simulink model "map_R2014a"  (R2014a)
settings: Solver=FixedStepDiscrete  StartTime=0  StopTime=300  FixedStep=0.5  RelTol=1e-3
PostLoadFcn:
  | , if any(exist('dsrtsu_mdlpostloadfcn', 'file') == [2, 3, 6]), try dsrtsu_mdlpostloadfcn('Execute', bdroot); catch fprintf('Error in PostLoadFcn (dsrtsu_mdlpostloadfcn) for model "%s":\n %s\n', bdroot, lasterr); end, end,
InitFcn:
  | load 'data/chi2_dat';
  | load 'data/innerLine_struct';
  | load 'data/middleLine_struct';
  | load 'data/outerLine_struct';
  | load 'data/innerLine';
  | load 'data/middleLine';
  | load 'data/outerLine';
  | load 'data/landmarks_patac_schimmel_ccw';
  | load 'data/patac_navi_array';
  | load 'data/sensor';
  | load 'data/map_struct';
  | addpath map_src
  | Integration_Parameter;
  | load 'TestData_001';
undefined symbols (not defined in the file or in its folder): chi2_dat, innerLine, landmarks_patac_schimmel_ccw, middleLine, outerLine, patac_navi_array
settings Model: DSRTSU_INTERNAL_RTI_VER=460  DSRTSU_INTERNAL_RTI_TYPE=rti1401  DSRTSU_INTERNAL_RTIFLEXRAYCONFIG=10  DSRTSU_INTERNAL_RTIFPGA=50  Creator=si8cwy  LastModifiedBy=Administrator
settings DataIOCC: SignalLoggingSaveFormat=ModelDataLogs
settings OptimizationCC: BlockReduction=off  ConditionallyExecuteInputs=off  OptimizeBlockIOStorage=off  BufferReuse=off  GlobalBufferReuse=off  ExpressionFolding=off  ExpressionDepthLimit=2147483647  LocalBlockOutputs=off  RollThreshold=100
settings DebuggingCC: MergeDetectMultiDrivingBlocksExec=error  MultiTaskDSMMsg=warning  MultiTaskCondExecSysMsg=none  FrameProcessingCompatibilityMsg=error  StateNameClashWarn=warning
settings HardwareCC: ProdIntDivRoundTo=Zero  ProdEndianess=BigEndian  ProdHWDeviceType=Generic->Custom  TargetIntDivRoundTo=Zero  TargetEndianess=BigEndian  TargetHWDeviceType=Generic->Custom
settings RTWCC: SystemTargetFile=rti1401.tlc  MakeCommand=make_rti  TemplateMakefile=rti1401.tmf  Description=dSPACE DS1401 Hardware Platform
settings STFCustomTargetCC: ParMdlRefBuildCompliant=on  ConcurrentExecutionCompliant=off  GeneratePreprocessorConditionals=Use local settings  SystemTargetFile=rti1401.tlc
settings GRTTargetCC: CompOptLevelCompliant=off  ConcurrentExecutionCompliant=off  GeneratePreprocessorConditionals=Use local settings  CombineOutputUpdateFcns=off  MatFileLogging=off  CPPClassGenCompliant=off  GRTInterface=on  ExtModeMexFile=noextcomm

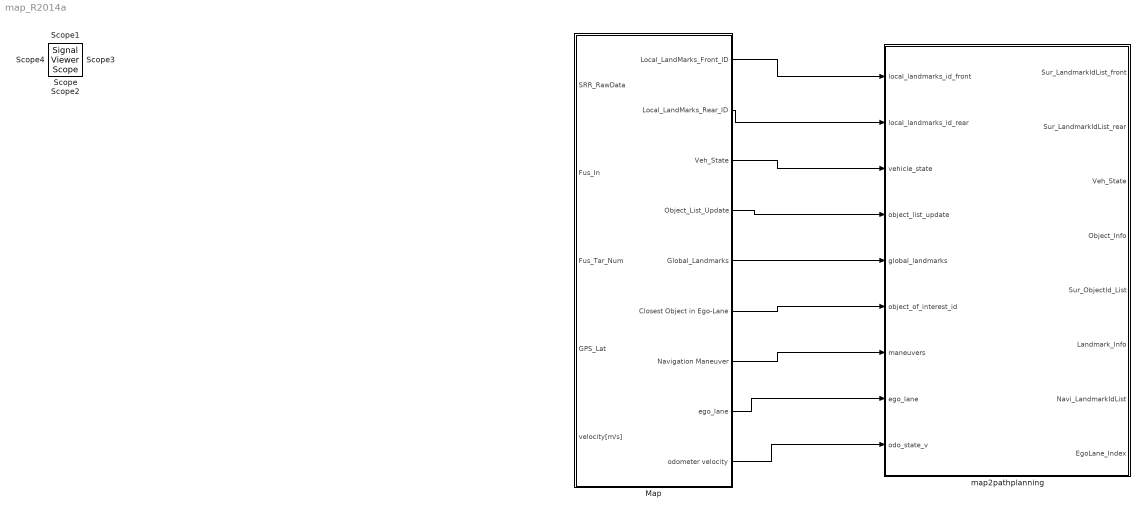
== system map_R2014a ==
  Map : Subsystem
  map2pathplanning : MATLAB Function  TreatAsAtomicUnit=on
      settings: PermitHierarchicalResolution=ParametersOnly
  Scope{,1..4} (5 alike) : SignalViewerScope  IOType=viewer  SampleTime=-1  ZoomMode=on
      Scope settings: TimeRange=auto  TickLabels=OneTimeTick  SaveToWorkspace=off  SaveName=ScopeData  YMin=-10  YMax=10  SampleInput=off
      Scope1 settings: TimeRange=auto  TickLabels=OneTimeTick  SaveToWorkspace=off  YMin=-10  YMax=10  SampleInput=off
      Scope2 settings: TimeRange=auto  TickLabels=OneTimeTick  SaveToWorkspace=off  SaveName=ScopeData2  YMin=-10  YMax=10  SampleInput=off
      Scope3 settings: TimeRange=auto  TickLabels=OneTimeTick  LimitDataPoints=on  SaveToWorkspace=off  SaveName=ScopeData3  YMin=-10  YMax=10  SampleInput=off
      Scope4 settings: TimeRange=auto  TickLabels=OneTimeTick  SaveToWorkspace=off  SaveName=ScopeData4  YMin=-10  YMax=10  SampleInput=off
  wires:
  Map/1(Local_LandMarks_Front_ID) -> map2pathplanning/1(local_landmarks_id_front)
  Map/3(Veh_State) -> map2pathplanning/3(vehicle_state)
  Map/4(Object_List_Update) -> map2pathplanning/4(object_list_update)
  Map/5("Global_Landmarks ") -> map2pathplanning/5(global_landmarks)
  Map/6(Closest Object in Ego-Lane) -> map2pathplanning/6(object_of_interest_id)
  Map/7(Navigation Maneuver) -> map2pathplanning/7(maneuvers)
  Map/9(odometer velocity) -> map2pathplanning/9(odo_state_v)
  Map/8(ego_lane) -> map2pathplanning/8(ego_lane)
  Map/2(Local_LandMarks_Rear_ID) -> map2pathplanning/2(local_landmarks_id_rear)

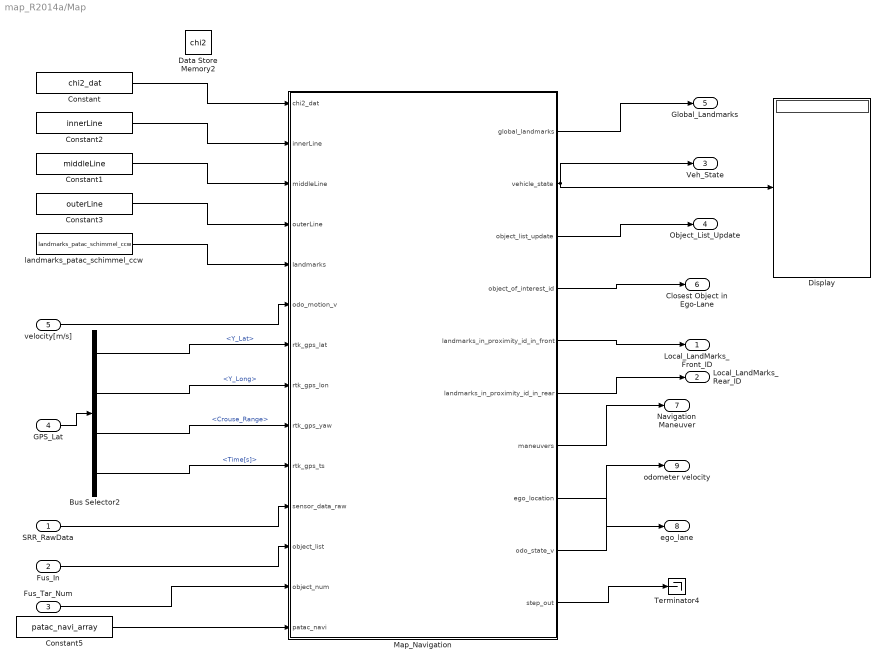
== system map_R2014a/Map ==
  SRR_RawData : Inport
  Fus_In : Inport  Port=2
  Fus_Tar_Num : Inport  Port=3
  GPS_Lat : Inport  Port=4
  velocity[m/s] : Inport  Port=5
  Bus Selector2 : BusSelector  OutputSignals=GPGLL.Y_Lat,GPGLL.Y_Long,GPHPR.Crouse_Range,GPGLL.Time[s]
  Constant : Constant  Value=chi2_dat
  Constant1 : Constant  Value=middleLine  OutDataTypeStr=Bus: middleLine_struct
  Constant2 : Constant  Value=innerLine  OutDataTypeStr=Bus: innerLine_struct
  Constant3 : Constant  Value=outerLine  OutDataTypeStr=Bus: outerLine_struct
  Constant5 : Constant  Value=patac_navi_array  OutDataTypeStr=double
  Data Store Memory2 : DataStoreMemory  DataStoreName=chi2  ReadBeforeWriteMsg=warning  WriteAfterWriteMsg=warning  WriteAfterReadMsg=warning  InitialValue=zeros(1,1000)  ShowAdditionalParam=off  OutDataTypeStr=double
  Display : Display
  Map_Navigation : MATLAB Function  TreatAsAtomicUnit=on
      settings: PermitHierarchicalResolution=ParametersOnly
  Terminator4 : Terminator
  landmarks_patac_schimmel_ccw : Constant  Value=landmarks_patac_schimmel_ccw  OutDataTypeStr=double
  Local_LandMarks_Front_ID : Outport
  Local_LandMarks_Rear_ID : Outport  Port=2
  Veh_State : Outport  Port=3
  Object_List_Update : Outport  Port=4
  "Global_Landmarks " : Outport  Port=5
  Closest Object in Ego-Lane : Outport  Port=6
  Navigation Maneuver : Outport  Port=7
  ego_lane : Outport  Port=8
  odometer velocity : Outport  Port=9
  wires:
  Map_Navigation/3(object_list_update) -> Object_List_Update/1
  Map_Navigation/2(vehicle_state) -> Veh_State/1, Display/1
  velocity[m/s]/1 -> Map_Navigation/6(odo_motion_v)
  GPS_Lat/1 -> Bus Selector2/1
  Bus Selector2/1 -> Map_Navigation/7(rtk_gps_lat)  "<Y_Lat>"
  Bus Selector2/2 -> Map_Navigation/8(rtk_gps_lon)  "<Y_Long>"
  Bus Selector2/3 -> Map_Navigation/9(rtk_gps_yaw)  "<Crouse_Range>"
  Bus Selector2/4 -> Map_Navigation/10(rtk_gps_ts)  "<Time[s]>"
  SRR_RawData/1 -> Map_Navigation/11(sensor_data_raw)
  Fus_In/1 -> Map_Navigation/12(object_list)
  Map_Navigation/4(object_of_interest_id) -> Closest Object in Ego-Lane/1
  Map_Navigation/7(maneuvers) -> Navigation Maneuver/1
  Constant/1 -> Map_Navigation/1(chi2_dat)
  Constant2/1 -> Map_Navigation/2(innerLine)
  Constant1/1 -> Map_Navigation/3(middleLine)
  Constant3/1 -> Map_Navigation/4(outerLine)
  landmarks_patac_schimmel_ccw/1 -> Map_Navigation/5(landmarks)
  Constant5/1 -> Map_Navigation/14(patac_navi)
  Map_Navigation/10(step_out) -> Terminator4/1
  Map_Navigation/9(odo_state_v) -> odometer velocity/1
  Map_Navigation/5(landmarks_in_proximity_id_in_front) -> Local_LandMarks_Front_ID/1
  Map_Navigation/1(global_landmarks) -> "Global_Landmarks "/1
  Map_Navigation/8(ego_location) -> ego_lane/1
  Map_Navigation/6(landmarks_in_proximity_id_in_rear) -> Local_LandMarks_Rear_ID/1
  Fus_Tar_Num/1 -> Map_Navigation/13(object_num)

== matlab function map_R2014a/Map/Map_Navigation ==
  data: global_landmarks output; vehicle_state output; object_list_update output; object_of_interest_id output; chi2_dat input; innerLine input; middleLine input; outerLine input; landmarks input; landmarks_in_proximity_id_in_front output [1..]; landmarks_in_proximity_id_in_rear output; odo_motion_v input; rtk_gps_lat input; rtk_gps_lon input; rtk_gps_yaw input; rtk_gps_ts input; sensor_data_raw input double size=[40 4]; object_list input double size=[127 26]; object_num input; chi2 data_store_memory; patac_navi input; maneuvers output; ego_location output; odo_state_v output; step_out output
%-------------------------------------------------------
% PATAC
% ADU
% SHD
% 
% Authors:  Binjian Xin
% Date   :  11-2016
%-------------------------------------------------------
% slam, explore data association algorithms
% hd_map: offline HD map orginal ground
% odo_motion: vehicle odometer data: odo_motion.x; odo_motion.y; odo_motion.yaw;
% sensor_data_raw: raw sensor data 40x4 [ID, x, y, MoveInfo]
% sensor_data_raw.srr[4] srr(1)-srr(4) are four SRR Radar raw data.
% srr(i).Measure --> [rho tita;...]
% srr(i).Rn --> [rho tita;...]c
% sensor_data_fusion: sensor fuison data; sensor_data_fusion
% 127x26
% [ID,RangeX,VelX,RangeY,VelY,MoveInfo,Width,Type,Fus_State,Confidence,
% P11,...P44]; FuseState Byte 9 for Lane Position Judge
% hd_map offline hd map, supposed to be converted to RTM 51r : wgs2utm(Lat,Lon,51,'N');
% hd_map.lanemarking1/lanemarking2/lanemarking3: three lanes, points in counterclockwise order; 1
% for left, 2 for middle, 3 for right;
% hd_map.landmark(:,5) (x,y,length, width, LandMarkType)
% rtk_gps: rtk_gps.[lat, lon, alt, yaw, pitch, roll, ts]
% 
% 
%   enumeration
%   XCrossing_Stop (11) % 十字路口停止线
%   XCrossing_Start (12) % 十字路口目标车道进入线
%   TCrossing_Stop (21)%T字路口停止线
%   TCrossing_Start (22)%T字路口目标车道进入线
%   ZCrossing (30)%人行横道线
%   Stop_1 (51)%边线1（沿车道横向边线）逆时针进入，摆渡车停车点。二号楼一号楼门口
%   Stop_2 (52)%边线2（沿车道横向边线）逆时针驶出
%   OL_LeftTurn_Stop (61)% 左转L形路口停止线，外道
%   OL_LeftTurn_Start (62)% 左转L形路口进入线，外道
%   RightTurn_Stop (71)% 右转L形路口停止线
%   RightTurn_Start (72)% 右转L形路口进入线
%   ParkSlotOnRoad_Stop (81)% 路上停车位边线1（沿车道横向边线）
%   ParkSlotOnRoad_Start (82)% 路上停车位边线2（沿车道横向边线）
%   ParkSlotOffRoad_Start (91)% 路边停车位边线1（沿车道横向边线）
%   ParkSlotOffRoad_Stop  (92)% 路边停车位边线2（沿车道横向边线）
%   RoadChange (100)% 车道宽度变化点，如两点间距离暗示车道宽度，则此时两点选取应保证，两点连线同测量处的车道垂直，或者增加车道宽度的域。
%   SpeedLimit (110)%限速标志，点类型
%   GroundArrow (120)%地上箭头（参考EPM3的箭头位置定义），点类型
%   TrafficLight (130)%交通灯位置，点类型
%   RoadChange (10)%车道宽度变化点
%   IL_LeftTurn_Stop (63)% 左转L形路口停止线，内道
%   IL_LeftTurn_Start (64)% 左转L形路口进入线，内道
%   UnClassified (180)%其他
%   end

%地标第六列属性：Unknown: 0， valid for inner lane: 1，valid for outer lane: 2，valid for both inner and outer lane: 3

%-------------------------------------------------------
%             t_in_utm,...
%             x_in_utm,...
%             y_in_utm,...
%             a_in_utm,...
%             delta_t,...
%             x_last,...
%             y_last,...
%             v_last,...
%             veh_ori_pos,...

function [global_landmarks,...
            vehicle_state, object_list_update, object_of_interest_id, ...
            landmarks_in_proximity_id_in_front, landmarks_in_proximity_id_in_rear,...
            maneuvers, ...
            ego_location, ...
            odo_state_v, ...
            step_out] ...
    = slam_ekf_patac_map_pose_output...
        (chi2_dat, ...
        innerLine, middleLine, outerLine, landmarks,...
        odo_motion_v,...
        rtk_gps_lat, rtk_gps_lon, rtk_gps_yaw, rtk_gps_ts, ...
        sensor_data_raw, object_list, object_num, patac_navi)
global chi2;
persistent step cnt veh_origin_pose configuration;
persistent x_in_utm_last y_in_utm_last a_in_utm_last t_in_utm_last a_rtk_offset veh_vel_last;
% local_landmarks_ids = zeros(200,1);

%Convert rtk raw data to longitude, latitude, yaw in radian and ts in
%second
[wgs_lat,wgs_lon,wgs_yaw,wgs_ts_in_sec] = rtkraw2wgs (rtk_gps_lat, rtk_gps_lon, rtk_gps_yaw,rtk_gps_ts);
[x_in_utm,y_in_utm,~,~] = wgs2utm(wgs_lat,wgs_lon,51,'N');
wgs_yaw = 2*pi - wgs_yaw;


%rtk system --> VCS offset
x_rtk_offset = 0;

y_rtk_offset = 0;
a_rtk_offset = 90*pi/180;%rtk calibration info input!
x_in_utm = x_in_utm+x_rtk_offset;
y_in_utm = y_in_utm+y_rtk_offset;
a_in_utm = wgs_yaw + a_rtk_offset;
t_in_utm = wgs_ts_in_sec;

if a_in_utm>2*pi
    a_in_utm = a_in_utm-2*pi;
end

chi2 = chi2_dat;

if  isempty(cnt)
    cnt = 1;
else
    cnt = cnt+1;
end

if (isempty(step) || cnt<100 )% first cycle
    step = 0;

    configuration = struct('ellipses',true,'tags',false,'odometry',true, ...
                            'noise',true,'alpha',0.99,'step_by_step',false,...
                            'people',false,'proximity',50, 'ground',1,'map',2,'observations',3,...
                            'compatibility',4,'ground_hypothesis',5,'hypothesis',6,...
                            'tables',7);
    configuration.step_by_step = true;   
    veh_origin_pose = struct('x_in_utm',0,'y_in_utm',0,'a_in_utm',0,'t_in_utm',0);   

    veh_origin_pose.x_in_utm = x_in_utm;% in Mercator
    veh_origin_pose.y_in_utm = y_in_utm;% in Mercator
    veh_origin_pose.a_in_utm = a_in_utm;
    veh_origin_pose.t_in_utm = t_in_utm;
    
    %Square One
    x_in_lcs = 0;
    y_in_lcs = 0;
    a_in_lcs = 0;
    t_in_lcs = 0;
    veh_pose = [0 0 0]';% x, y, yaw in LCS
    %standing still
    veh_vel = [0 0]';% V_x, V_y in LCS
    vehicle_state = [veh_pose; veh_vel];

    x_in_utm_last = x_in_utm;
    y_in_utm_last = y_in_utm;
    a_in_utm_last = a_in_utm;
    t_in_utm_last = t_in_utm;

%     a_last = a_in_utm;
    veh_vel_last = [0 0]';

    landmarks_in_proximity_id_in_front = zeros(size(landmarks,1),1);
    landmarks_in_proximity_id_in_rear  = zeros(size(landmarks,1),1); 
    maneuvers = patac_navi;
    global_landmarks = landmarks;
    odo_state_v = odo_motion_v;
    step_out = 0;
    object_list_update = object_list;
    object_of_interest_id = 0;
    ego_location = -1; % due to invalid data from rtk ego locatoin cannot be determined.
    delta_t = 0;
    
    x_last = 0;
    y_last = 0;
    v_last = [0;0];
    veh_ori_pos = [veh_origin_pose.x_in_utm;veh_origin_pose.y_in_utm;veh_origin_pose.a_in_utm;veh_origin_pose.t_in_utm];

    return;

else %after first cycle    
    step = step +1;
    if(abs(rtk_gps_lat)<1e-6 ...
       || abs(rtk_gps_lon)<1e-6 ...
       || abs(rtk_gps_ts)<1e-6...
       )%if invalid rtk data after initialization halfways due to rtk signal loss
        t_in_lcs = (t_in_utm_last +0.01)-veh_origin_pose.t_in_utm;
        x_in_lcs = (x_in_utm_last+veh_vel_last(1)*0.01)-veh_origin_pose.x_in_utm;
        y_in_lcs = (y_in_utm_last+veh_vel_last(2)*0.01)-veh_origin_pose.y_in_utm;
        a_in_lcs = a_in_utm_last;
        veh_vel = veh_vel_last; 
    elseif(abs(wgs_ts_in_sec - t_in_utm_last)<1e-6)
        t_in_lcs = (t_in_utm_last +0.01)-veh_origin_pose.t_in_utm;
        x_in_lcs = (x_in_utm_last+veh_vel_last(1)*0.01)-veh_origin_pose.x_in_utm;
        y_in_lcs = (y_in_utm_last+veh_vel_last(2)*0.01)-veh_origin_pose.y_in_utm;
        a_in_lcs = a_in_utm_last;
        veh_vel = veh_vel_last; 
    else
        t_in_lcs = t_in_utm - veh_origin_pose.t_in_utm;
        x_in_lcs = x_in_utm-veh_origin_pose.x_in_utm;
        y_in_lcs = y_in_utm-veh_origin_pose.y_in_utm;
        a_in_lcs = a_in_utm; %a_in_utm - veh_origin_pose.a_in_utm;
        %veh_vel = [(x_in_lcs-x_in_lcs_last)/0.01; (y_in_lcs-y_in_lcs_last)/0.01];%(ts_in_lcs - ts_in_lcs_last);
        veh_vel = [0;0];
        veh_vel(1) = (x_in_utm-x_in_utm_last)*100;%(x_in_lcs-x_in_lcs_last)*100;
        veh_vel(2) = (y_in_utm-y_in_utm_last)*100;%(y_in_lcs-y_in_lcs_last)*100;%(ts_in_lcs - ts_in_lcs_last);
    end

    delta_t = (t_in_utm - t_in_utm_last);
    
    x_last = x_in_utm_last;
    y_last = y_in_utm_last;
    v_last = veh_vel_last;
    veh_ori_pos = [veh_origin_pose.x_in_utm;veh_origin_pose.y_in_utm;veh_origin_pose.a_in_utm;veh_origin_pose.t_in_utm];
    
    veh_pose = [x_in_lcs y_in_lcs a_in_lcs]';% x, y, yaw in LCS
    vehicle_state = [veh_pose; veh_vel];

    x_in_utm_last = x_in_utm;
    y_in_utm_last = y_in_utm;
    a_in_utm_last = a_in_utm;

%     a_last = a_in_utm;
    t_in_utm_last = t_in_utm;
    veh_vel_last = veh_vel;
end

%{
if isempty(step)
    step = 0;
    
    configuration = struct('ellipses',true,'tags',false,'odometry',true, ...
                            'noise',true,'alpha',0.99,'step_by_step',false,...
                            'people',false,'proximity',50, 'ground',1,'map',2,'observations',3,...
                            'compatibility',4,'ground_hypothesis',5,'hypothesis',6,...
                            'tables',7);
    configuration.step_by_step = true;                
    veh_origin_pose = struct('x_in_utm',0,'y_in_utm',0,'a_in_utm',0,'t_in_utm',0);   

    veh_origin_pose.x_in_utm = x_in_utm;% in Mercator
    veh_origin_pose.y_in_utm = y_in_utm;% in Mercator
    veh_origin_pose.a_in_utm = a_in_utm;
    veh_origin_pose.t_in_utm = t_in_utm;
    
    %Square One
    x_in_lcs = 0;
    y_in_lcs = 0;
    a_in_lcs = 0;
%   t_in_lcs = 0;
    veh_pose = [0 0 0]';% x, y, yaw in LCS
    %standing still
    veh_vel = [0 0]';% V_x, V_y in LCS
    vehicle_state = [veh_pose; veh_vel];
    
    x_in_utm_last = x_in_utm;
    y_in_utm_last = y_in_utm;
    a_in_utm_last = a_in_utm;
    t_in_utm_last = t_in_utm;
    veh_vel_last = [0 0]';

    landmarks_in_proximity_id_in_front = zeros(size(landmarks,1),1);
    landmarks_in_proximity_id_in_rear  = zeros(size(landmarks,1),1); 
    maneuvers = patac_navi;
    global_landmarks = landmarks;
    odo_state_v = odo_motion_v;
    step_out = 0;
    object_list_update = object_list;
    object_of_interest_id = 0;
    ego_location = -1; % due to invalid data from rtk ego locatoin cannot be determined.
    return;         
%{
%     delta_t = 0;
%     x_last = x_in_utm_last;
%     y_last = y_in_utm_last;
%     v_last = veh_vel_last;
%     veh_ori_pos = [veh_origin_pose.x_in_utm;veh_origin_pose.y_in_utm;veh_origin_pose.a_in_utm;veh_origin_pose.t_in_utm];
    
%     if(~(abs(rtk_gps_lat)<1e-6 || abs(rtk_gps_lon)<1e-6 || abs(rtk_gps_ts)<1e-6))
%         %valid rtk signal on first cycle
%         step = 1;
%     else%invalid rtk on first cycle
%     end        
%}
else %after first cycle  
    if( step ==0 )%initialisation
        if(abs(rtk_gps_lat)<1e-6 ...
           || abs(rtk_gps_lon)<1e-6 ...
           || abs(rtk_gps_ts)<1e-6...
          )
            % invalid rtk after first cycle
            step = 0;
            veh_pose = [0 0 0]';% x, y, yaw in LCS
            %standing still
            veh_vel = [0 0]';% V_x, V_y in LCS
            vehicle_state = [veh_pose; veh_vel];
            
            landmarks_in_proximity_id_in_front = zeros(size(landmarks,1),1);
            landmarks_in_proximity_id_in_rear  = zeros(size(landmarks,1),1); 
            maneuvers = patac_navi;
            global_landmarks = landmarks;
            odo_state_v = odo_motion_v;
            step_out = 0;
            object_list_update = object_list;
            object_of_interest_id = 0;
            ego_location = -1;% due to invalid data from rtk ego locatoin cannot be determined.
%             delta_t = 0;
%             x_last = x_in_utm_last;
%             y_last = y_in_utm_last;
%             v_last = veh_vel_last;
%             veh_ori_pos = [veh_origin_pose.x_in_utm;veh_origin_pose.y_in_utm;veh_origin_pose.a_in_utm;veh_origin_pose.t_in_utm];
            return;
        else% valid rtk after first cycle for initialization, initialization most probably in this branch
            step = 1;

            veh_origin_pose.x_in_utm = x_in_utm;% in Mercator
            veh_origin_pose.y_in_utm = y_in_utm;% in Mercator
            veh_origin_pose.a_in_utm = a_in_utm;
            veh_origin_pose.t_in_utm = t_in_utm;
            
            x_in_lcs = 0;
            y_in_lcs = 0;
            a_in_lcs = a_in_utm;
%           t_in_lcs = wgs_ts_in_sec - veh_origin_pose.t_in_utm;
            veh_vel =  [0 0]';%[x_in_lcs-x_in_lcs_last; y_in_lcs-y_in_lcs_last]/(ts_in_lcs - ts_in_lcs_last);
            veh_pose = [x_in_lcs y_in_lcs a_in_lcs]';% x, y, yaw in LCS
            vehicle_state = [veh_pose; veh_vel];
%             delta_t = 0;
%             x_last = x_in_utm_last;
%             y_last = y_in_utm_last;
%             v_last = veh_vel_last;
%             veh_ori_pos = [veh_origin_pose.x_in_utm;veh_origin_pose.y_in_utm;veh_origin_pose.a_in_utm;veh_origin_pose.t_in_utm];

            x_in_utm_last = x_in_utm;
            y_in_utm_last = y_in_utm;
            a_in_utm_last = a_in_utm;
            t_in_utm_last = t_in_utm;
            veh_vel_last = [0 0]';  
            
            landmarks_in_proximity_id_in_front = zeros(size(landmarks,1),1);
            landmarks_in_proximity_id_in_rear  = zeros(size(landmarks,1),1); 
            maneuvers = patac_navi;
            global_landmarks = landmarks;
            odo_state_v = odo_motion_v;
            step_out = 0;
            object_list_update = object_list;
            object_of_interest_id = 0;
            ego_location = -1; % due to invalid data from rtk ego locatoin cannot be determined.
            return;         
        end
    else% after initialization

        step = step +1;
        if(abs(rtk_gps_lat)<1e-6 ...
           || abs(rtk_gps_lon)<1e-6 ...
           || abs(rtk_gps_ts)<1e-6...
           )%if invalid rtk data after initialization halfways due to rtk signal loss
%             t_in_lcs = (t_in_utm_last +0.01)-veh_origin_pose.t_in_utm;
            x_in_lcs = (x_in_utm_last+veh_vel_last(1)*0.01)-veh_origin_pose.x_in_utm;
            y_in_lcs = (y_in_utm_last+veh_vel_last(2)*0.01)-veh_origin_pose.y_in_utm;
            a_in_lcs = a_in_utm_last;
            veh_vel = veh_vel_last; 
            
            x_in_utm_last = x_in_utm_last+veh_vel_last(1)*0.01;
            y_in_utm_last = y_in_utm_last+veh_vel_last(2)*0.01;
%             a_in_utm_last = a_in_utm_last;
            t_in_utm_last = t_in_utm+0.01;
            veh_vel_last = veh_vel;            
        elseif(abs(wgs_ts_in_sec - t_in_utm_last)<1e-6)
    %         t_in_lcs = (t_in_utm_last +0.01)-veh_origin_pose.t_in_utm;
            x_in_lcs = (x_in_utm_last+veh_vel_last(1)*0.01)-veh_origin_pose.x_in_utm;
            y_in_lcs = (y_in_utm_last+veh_vel_last(2)*0.01)-veh_origin_pose.y_in_utm;
            a_in_lcs = a_in_utm_last;
            veh_vel = veh_vel_last; 
            x_in_utm_last = x_in_utm_last+veh_vel_last(1)*0.01;
            y_in_utm_last = y_in_utm_last+veh_vel_last(2)*0.01;
%             a_in_utm_last = a_in_utm_last;
            t_in_utm_last = t_in_utm+0.01;
            veh_vel_last = veh_vel;                 
        else
%             t_in_lcs = t_in_utm - veh_origin_pose.t_in_utm;
            x_in_lcs = x_in_utm-veh_origin_pose.x_in_utm;
            y_in_lcs = y_in_utm-veh_origin_pose.y_in_utm;
            a_in_lcs = a_in_utm; %a_in_utm - veh_origin_pose.a_in_utm;
%             veh_vel = [(x_in_utm-x_in_utm_last)/0.01; (y_in_utm-y_in_utm_last)/0.01];%(ts_in_lcs - ts_in_lcs_last);
            veh_vel = [(x_in_utm-x_in_utm_last); (y_in_utm-y_in_utm_last)]/(t_in_utm - t_in_utm_last);
%             veh_vel_norm = norm(veh_vel),
%             odo_motion_v,
%             dev=(veh_vel_norm-odo_motion_v)/odo_motion_v,
%             veh_vel = [0;0];
%             veh_vel(1) = (x_in_utm-x_in_utm_last)*100;%(x_in_lcs-x_in_lcs_last)*100;
%             veh_vel(2) = (y_in_utm-y_in_utm_last)*100;%(y_in_lcs-y_in_lcs_last)*100;%(ts_in_lcs - ts_in_lcs_last);
            x_in_utm_last = x_in_utm;
            y_in_utm_last = y_in_utm;
            a_in_utm_last = a_in_utm;
            t_in_utm_last = t_in_utm;
            veh_vel_last = veh_vel;        
        end

%         delta_t = (t_in_utm - t_in_utm_last);
%         x_last = x_in_utm_last;
%         y_last = y_in_utm_last;
%         v_last = veh_vel_last;
%         veh_ori_pos = [veh_origin_pose.x_in_utm;veh_origin_pose.y_in_utm;veh_origin_pose.a_in_utm;veh_origin_pose.t_in_utm];
% 
        veh_pose = [x_in_lcs y_in_lcs a_in_lcs]';% x, y, yaw in LCS
        vehicle_state = [veh_pose; veh_vel];
    end
end
%}

%relocate lane markings in LCS, origin is the starting point.
innerLine.coordinate = innerLine.coordinate - ...
 [ones(size(innerLine.coordinate,1),1).*veh_origin_pose.x_in_utm,...
  ones(size(innerLine.coordinate,1),1).*veh_origin_pose.y_in_utm];
middleLine.coordinate = middleLine.coordinate - ...
 [ones(size(middleLine.coordinate,1),1).*veh_origin_pose.x_in_utm,...
  ones(size(middleLine.coordinate,1),1).*veh_origin_pose.y_in_utm];
outerLine.coordinate = outerLine.coordinate - ...
 [ones(size(outerLine.coordinate,1),1).*veh_origin_pose.x_in_utm,...
  ones(size(outerLine.coordinate,1),1).*veh_origin_pose.y_in_utm];

%relocate landmarks in LCS, origin is the starting point.
landmarks(:,1) = landmarks(:,1) - veh_origin_pose.x_in_utm;% landmarks in LCS!
landmarks(:,2) = landmarks(:,2) - veh_origin_pose.y_in_utm;% landmarks in LCS!
landmarks(:,3) = landmarks(:,3) - veh_origin_pose.x_in_utm;% landmarks in LCS!
landmarks(:,4) = landmarks(:,4) - veh_origin_pose.y_in_utm;% landmarks in LCS!

%relocate navigation maneuver list in LCS, origin is the starting point.
patac_navi(:,1) = patac_navi(:,1) - veh_origin_pose.x_in_utm;%navigation maneuver in LCS!
patac_navi(:,2) = patac_navi(:,2) - veh_origin_pose.y_in_utm;%navigation maneuver in LCS!

% plot ground
if(step==1)
    draw_map_nav_ground(innerLine.coordinate,innerLine.Vertex_index,...
                      middleLine.coordinate,middleLine.Vertex_index,...
                      outerLine.coordinate,outerLine.Vertex_index,...
                      landmarks, vehicle_state, patac_navi, configuration);
end
% % pause


%Relocate object list in LCS
%SCS --> VCS offset 
x_scs_offset = -5.24/2.0;%vehicle length 5.24m
y_scs_offset = 0;%vehicle width 1.8m

%VCS --> CCS (Control Coordinate System) offset 
x_ccs_offset = 0;
y_ccs_offset = 0;
% x_offset = x_scs_offset+x_ccs_offset;
% y_offset = y_scs_offset+y_ccs_offset;


object_loc = [object_list(1:object_num,2),object_list(1:object_num,4)]';
Tab = [ x_scs_offset + x_in_lcs; y_scs_offset + y_in_lcs; a_in_lcs];
Pa = tpcomp(Tab, object_loc);
object_list(1:object_num,2)=Pa(1,:)';%object_list(:,2)+ x_scs_offset + x_in_lcs;%RangeX in LCS, displacement of VCS to SCS by 2.6m, half of vehicle length
object_list(1:object_num,4)=Pa(2,:)';%object_list(:,4)+ y_scs_offset + y_in_lcs;%RangeY in LCS

object_vec = [object_list(1:object_num,3),object_list(1:object_num,5)]';
Tab = [ veh_vel(1); veh_vel(2); a_in_lcs];
Pb = tpcomp(Tab, object_vec);
object_list(1:object_num,3)=Pb(1,:)';%object_list(:,3)+ veh_vel(1);%VelX
object_list(1:object_num,5)=Pb(2,:)';%object_list(:,5)+ veh_vel(2);%VelY    

raw_loc = [sensor_data_raw(:,2),sensor_data_raw(:,3)]';
Tab = [ x_scs_offset + x_in_lcs; y_scs_offset + y_in_lcs; a_in_lcs];
Pa = tpcomp(Tab, raw_loc);
sensor_data_raw(:,2)=Pa(1,:)';%object_list(:,2)+ x_scs_offset + x_in_lcs;%RangeX in LCS, displacement of VCS to SCS by 2.6m, half of vehicle length
sensor_data_raw(:,3)=Pa(2,:)';%object_list(:,4)+ y_scs_offset + y_in_lcs;%RangeY in LCS

%find local landmarks
option.firstTime=1;
option.clockWise=0;  %0 for counter-clockwise，1 for clockwise    
[landmarks_in_proximity_id_in_front, landmarks_in_proximity_id_in_rear] = quest_map4landmark (x_in_lcs, y_in_lcs, landmarks,middleLine.coordinate, middleLine.Vertex_index,configuration,option);

%     sensor_data_raw(:,2)=sensor_data_raw(:,2)+ x0_offset + veh_origin_pose.x;%RangeX, displacement of VCS to SCS by 2.6m, half of vehicle length
%     sensor_data_raw(:,3)=sensor_data_raw(:,3)+ y0_offset + veh_origin_pose.y;%RangeY

%    [veh_pose, veh_vel] = slam_ekf_patac (inner, middle, outer, landmarks, ...
%         odo_motion_x, odo_motion_y, odo_motion_yaw, ...

%         rtk_gps_lat, rtk_gps_lon, rtk_gps_yaw, rtk_gps_ts, ...
%         sensor_data_raw,...
%         proximity);
   
%locate objects in lanes    
%decide object list location in lanes
object_list_update  = object_localization(object_list, object_num, innerLine.coordinate,innerLine.Vertex_index,...
                                                      middleLine.coordinate,middleLine.Vertex_index,...
                                                      outerLine.coordinate,outerLine.Vertex_index,...
                                                      option);
%find the closest object in ego lane (probably CIPV)
[obj_closest_in_path_ID, ~,ego_location] = objects_of_interest(object_list_update,object_num,...
    x_in_lcs, y_in_lcs, innerLine.coordinate, innerLine.Vertex_index,...
    middleLine.coordinate, middleLine.Vertex_index,...
    outerLine.coordinate, outerLine.Vertex_index, option);
object_of_interest_id = obj_closest_in_path_ID;

maneuvers = patac_navi;
global_landmarks = landmarks;
odo_state_v = odo_motion_v;
step_out = step;

% draw_map_nav_ground (innerLine.coordinate,innerLine.Vertex_index,...
%                       middleLine.coordinate,middleLine.Vertex_index,...
%                       outerLine.coordinate,outerLine.Vertex_index,...
%                       landmarks, configuration);

draw_observations_nav_ground(innerLine.coordinate, innerLine.Vertex_index,...
                                middleLine.coordinate, middleLine.Vertex_index,...
                                outerLine.coordinate, outerLine.Vertex_index,...
                                landmarks, landmarks_in_proximity_id_in_front, ...
                                landmarks_in_proximity_id_in_rear, vehicle_state, object_list, ...
                                object_of_interest_id, sensor_data_raw, ...
                                patac_navi,configuration);

== matlab function map_R2014a/map2pathplanning ==
  data: local_landmarks_id_front input; local_landmarks_id_rear input; vehicle_state input; object_list_update input; global_landmarks input; object_of_interest_id input; maneuvers input; ego_lane input; odo_state_v input; Sur_LandmarkIdList_front output; Sur_LandmarkIdList_rear output; Veh_State output; Object_Info output; Sur_ObjectId_List output; Landmark_Info output; Navi_LandmarkIdList output; EgoLane_Index output
function [Sur_LandmarkIdList_front,...
          Sur_LandmarkIdList_rear,...
          Veh_State,...
          Object_Info,...
          Sur_ObjectId_List,...
          Landmark_Info,...
          Navi_LandmarkIdList,...
          EgoLane_Index]  = ...
    map2pp(local_landmarks_id_front,...
            local_landmarks_id_rear,...
            vehicle_state,...
            object_list_update, ...
            global_landmarks,...
            object_of_interest_id, ...
            maneuvers, ...
            ego_lane, ...
            odo_state_v)
        
        Sur_LandmarkIdList_front = local_landmarks_id_front;
        Sur_LandmarkIdList_rear = local_landmarks_id_rear;
        Object_Info = object_list_update;
        Landmark_Info = global_landmarks;
           
        Veh_State = zeros(1,8);
        Veh_State(1:5) = vehicle_state';
        Veh_State(8) = odo_state_v;
        Navi_LandmarkIdList = maneuvers;

        Sur_ObjectId_List = zeros(3,10);
        Sur_ObjectId_List(1,1) = object_of_interest_id;
        
        EgoLane_Index = ego_lane;
% %     %#codegen
%     OperationFinishFlg = 1;
%     Landmark_Info = zeros(30,5);
% %     Landmark_Info(1,:) = [0,0,0,-4,12];Landmark_Info(8,:) = [0,0,-4,0,11];
% %     Landmark_Info(2,:) = [100,0,100,-4,11];Landmark_Info(3,:) = [100,0,104,0,12];
% %     Landmark_Info(4,:) = [100,100,104,100,11];Landmark_Info(5,:) = [100,100,100,104,12];
% %     Landmark_Info(6,:) = [0,100,0,104,11];Landmark_Info(7,:) = [0,100,-4,100,12];
% %     for i = 1:8 
% %         plot(Landmark_Info(i,1),Landmark_Info(i,2),'*',Landmark_Info(i,3),Landmark_Info(i,4),'*');
% %         hold on        
% %     end
%     Landmark_Info(1,:) = [0,0,0,-4,12];Landmark_Info(8,:) = [-20,20,-24,20,11];
%     Landmark_Info(2,:) = [100,0,100,-4,11];Landmark_Info(3,:) = [120,20,124,20,12];
%     Landmark_Info(4,:) = [120,120,124,120,11];Landmark_Info(5,:) = [100,140,100,144,12];
%     Landmark_Info(6,:) = [0,140,0,144,11];Landmark_Info(7,:) = [-20,120,-24,120,12];
%     Navi_LandmarkIdList = [0,20,40,2;100,20,40,2;100,120,40,2;0,120,40,2];
%     EgoLane_Index = 1;
%     Veh_State = [99.5,-2,0,0,0,0,0,0]';
%     Sur_ObjectId_List = zeros(3,10);
%     Sur_ObjectId_List(1,:) = [1,2,0,0,0,0,0,0,0,0];
%     Object_Info = zeros(127,26);
%     Object_Info(1,:) = [1,122,0,50,0,1,2.5,0,0,0,0,0,0,0,0,0,1,30,10,0,0,1,2.5,0,0,0;];    
%     Object_Info(2,:) = [2,122,0,-50,0,1,2.5,0,0,0,0,0,0,0,0,0,1,30,10,0,0,1,2.5,0,0,0;]; 
%     Object_Info(3,:) = [3,30,10,0,0,1,2.5,0,0,0,0,0,0,0,0,0,1,30,10,0,0,1,2.5,0,0,0;];    
%     Object_Info(4,:) = [4,30,10,0,0,1,2.5,0,0,0,0,0,0,0,0,0,1,30,10,0,0,1,2.5,0,0,0;]; 
%     Sur_LandmarkIdList_front = [2,3,4,5,6,7,8,1,0]';
%     Sur_LandmarkIdList_rear = [2,3,4,5,6,7,8,1,0]';
end
